simulink model "Zlinearyzowany"  (R2017a)
settings: Solver=FixedStepAuto  StartTime=0.0  StopTime=150  FixedStep=0.1  RelTol=1e-3  EnableMultiTasking=on
values from neighbouring files (symbols this model uses):
  A = pi*R1*R1    (= 10.9999393421)    [Lab2.m]    (also in ModelDataNonlinear.m)
  B = (pi*R2*R2)/(3*H2*H2)    (= 0.00337009933323)    [Lab2.m]    (also in Lab8.m = deltah20max / k; Lab9.m = 0.4; ModelDataNonlinear.m)
  C1 = 1.372    [Lab2.m]    (also in ModelDataNonlinear.m)
  C2 = 0.332756    [Lab2.m]    (also in ModelDataNonlinear.m)
  deltaw = deltaq1    [Lab2.m]    (also in Lab3.m = 0; Lab8.m = deltah20max / 3; ModelDataNonlinear.m = 0.1*w0)
  h10 = (q10/C1).^2    [Lab2.m]    (also in ModelDataNonlinear.m)
  h20 = h2max/2    (= 8)    [Lab2.m]    (also in ModelDataNonlinear.m)
  k = 5    [Lab1.m]    (also in Lab2.m = (2*sqrt(h20))/C2; ModelData.m = 17)
  kr = 1.84/2    (= 0.92)    [Lab1.m]    (also in Lab4.m = 0.95*T/(k*T0); Lab7.m = 0.0803; Lab9.m = 0.0679)
  q10 = C2*sqrt(h20)    [Lab2.m]    (also in ModelDataNonlinear.m)
  T1 = 3    [Lab1.m]    (also in Lab2.m = 2*pi*R1*R1*sqrt(h10)/C1; ModelData.m = 10.998)
  T2 = 4    [Lab1.m]    (also in Lab2.m = 2*A*sqrt(h10)/C1; ModelData.m = 10.998)
  T3 = 8    [Lab1.m]    (also in Lab3.m = 0.5*T1; Lab4.m = 0.5 * T1; ModelData.m = min(T1, T2) / 2)
  Td = 0.42*T0    [Lab4.m]
  Tf = 0.05 * Td    (= 0.19375)    [Lab4.m]
  Ti = 2.4*T0    [Lab4.m]    (also in Lab9.m = 17.823)
settings Model: Creator=Ganofir  LastModifiedBy=ishiguro
settings DataIOCC: SaveFormat=Array
settings OptimizationCC: LifeSpan=inf
settings DebuggingCC: ModelReferenceDataLoggingMessage=none  SFUnexpectedBacktrackingDiag=warning  SFNoUnconditionalDefaultTransitionDiag=warning  SFExecutionAtInitializationDiag=none
settings HardwareCC: ProdBitPerPointer=32  ProdBitPerSizeT=32  ProdBitPerPtrDiffT=32  ProdLargestAtomicFloat=None  ProdIntDivRoundTo=Undefined  ProdEndianess=Unspecified  ProdWordSize=32  ProdHWDeviceType=32-bit Generic
settings ModelReferenceCC: PropagateSignalLabelsOutOfModel=off
settings GRTTargetCC: TargetLangStandard=C89/C90 (ANSI)  GeneratePreprocessorConditionals=Disable all
settings ConfigComp: CovMetricSettings=dw  CovHtmlReporting=on  CovSaveCumulativeToWorkspaceVar=on  CovSaveSingleToWorkspaceVar=on  CovExternalEMLEnable=off

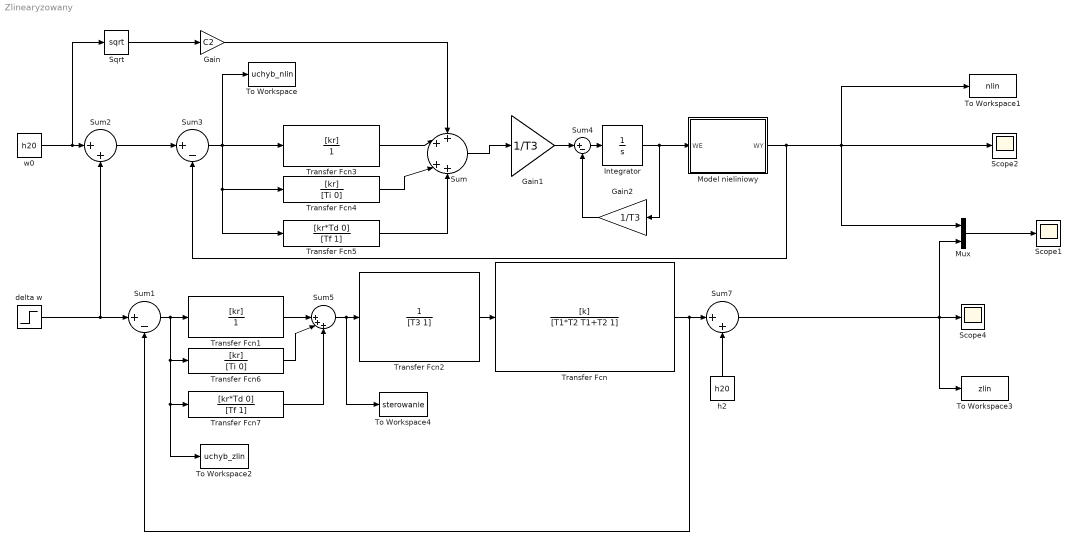
== system Zlinearyzowany ==
  Gain : Gain  Gain=C2
  Gain1 : Gain  Gain=1/T3
  Gain2 : Gain  Gain=1/T3
  Integrator : Integrator  InitialCondition=q10
  Model nieliniowy : Subsystem
  Mux : Mux  Inputs=2
  Scope1 : Scope
  Scope2 : Scope
  Scope4 : Scope
  Sqrt : Sqrt  SaturateOnIntegerOverflow=on
  Sum : Sum  Inputs=++|++
  Sum1 : Sum  Inputs=|+-
  Sum2 : Sum  Inputs=|++
  Sum3 : Sum  Inputs=|+-
  Sum4 : Sum  Inputs=|+-
  Sum5 : Sum  Inputs=||+++
  Sum7 : Sum  Inputs=|++
  To Workspace : ToWorkspace  VariableName=uchyb_nlin  SampleTime=-1
  To Workspace1 : ToWorkspace  VariableName=nlin  SampleTime=-1
  To Workspace2 : ToWorkspace  VariableName=uchyb_zlin  SampleTime=-1
  To Workspace3 : ToWorkspace  VariableName=zlin  SampleTime=-1
  To Workspace4 : ToWorkspace  VariableName=sterowanie  SampleTime=-1
  Transfer Fcn : TransferFcn  Numerator=[k]  Denominator=[T1*T2 T1+T2 1]
  Transfer Fcn1 : TransferFcn  Numerator=[kr]  Denominator=[1]
  Transfer Fcn2 : TransferFcn  Denominator=[T3 1]
  Transfer Fcn3 : TransferFcn  Numerator=[kr]  Denominator=[1]
  Transfer Fcn4 : TransferFcn  Numerator=[kr]  Denominator=[Ti 0]
  Transfer Fcn5 : TransferFcn  Numerator=[kr*Td 0]  Denominator=[Tf 1]
  Transfer Fcn6 : TransferFcn  Numerator=[kr]  Denominator=[Ti 0]
  Transfer Fcn7 : TransferFcn  Numerator=[kr*Td 0]  Denominator=[Tf 1]
  delta w : Step  Time=0  After=deltaw  SampleTime=0
  h2 : Constant  Value=h20
  w0 : Constant  Value=h20
  wires:
  delta w/1 -> Sum1/1, Sum2/2
  Sum7/1 -> Mux/2, To Workspace3/1, Scope4/1
  h2/1 -> Sum7/2
  Transfer Fcn/1 -> Sum1/2, Sum7/1
  Transfer Fcn2/1 -> Transfer Fcn/1
  Sum1/1 -> Transfer Fcn6/1, Transfer Fcn7/1, To Workspace2/1, Transfer Fcn1/1
  Mux/1 -> Scope1/1
  w0/1 -> Sqrt/1, Sum2/1
  Sum2/1 -> Sum3/1
  Sum3/1 -> Transfer Fcn4/1, Transfer Fcn5/1, To Workspace/1, Transfer Fcn3/1
  Integrator/1 -> Gain2/1, Model nieliniowy/1(WE)
  Model nieliniowy/1(WY) -> Sum3/2, To Workspace1/1, Scope2/1, Mux/1
  Sum/1 -> Gain1/1
  Transfer Fcn3/1 -> Sum/2
  Sqrt/1 -> Gain/1
  Gain/1 -> Sum/1
  Gain1/1 -> Sum4/1
  Sum4/1 -> Integrator/1
  Gain2/1 -> Sum4/2
  Transfer Fcn5/1 -> Sum/4
  Transfer Fcn4/1 -> Sum/3
  Transfer Fcn7/1 -> Sum5/3
  Transfer Fcn6/1 -> Sum5/2
  Transfer Fcn1/1 -> Sum5/1
  Sum5/1 -> To Workspace4/1, Transfer Fcn2/1

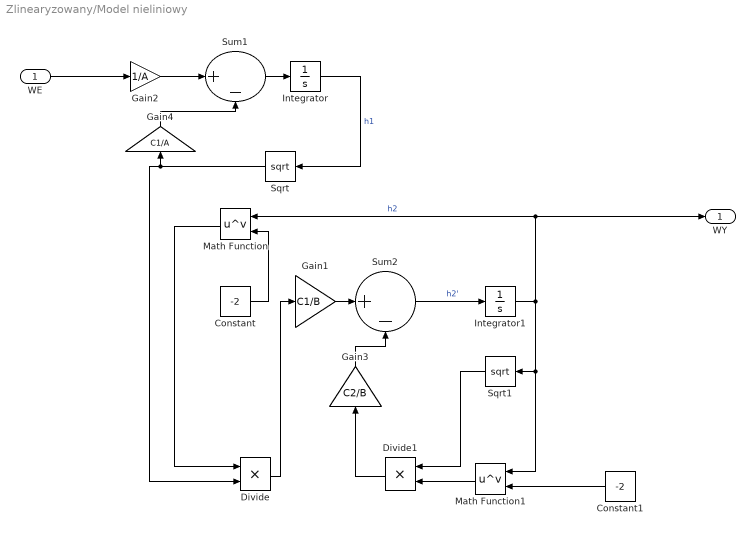
== system Zlinearyzowany/Model nieliniowy ==
  WE : Inport
  Constant : Constant  Value=-2
  Constant1 : Constant  Value=-2
  Divide : Product  Inputs=**
  Divide1 : Product  Inputs=**
  Gain1 : Gain  Gain=C1/B
  Gain2 : Gain  Gain=1/A
  Gain3 : Gain  Gain=C2/B
  Gain4 : Gain  Gain=C1/A
  Integrator : Integrator  InitialCondition=h10
  Integrator1 : Integrator  InitialCondition=h20
  Math Function : Math  Operator=pow  SaturateOnIntegerOverflow=on
  Math Function1 : Math  Operator=pow  SaturateOnIntegerOverflow=on
  Sqrt : Sqrt  SaturateOnIntegerOverflow=on
  Sqrt1 : Sqrt  SaturateOnIntegerOverflow=on
  Sum1 : Sum  Inputs=|+-
  Sum2 : Sum  Inputs=|+-
  WY : Outport
  wires:
  Sum1/1 -> Integrator/1
  Sqrt1/1 -> Divide1/1
  Gain4/1 -> Sum1/2
  Integrator1/1 -> Math Function/1, WY/1, Math Function1/1, Sqrt1/1  "h2"
  Sqrt/1 -> Divide/2, Gain4/1
  Gain3/1 -> Sum2/2
  Sum2/1 -> Integrator1/1  "h2'"
  Divide1/1 -> Gain3/1
  Integrator/1 -> Sqrt/1  "h1"
  Gain1/1 -> Sum2/1
  Divide/1 -> Gain1/1
  Gain2/1 -> Sum1/1
  WE/1 -> Gain2/1
  Constant/1 -> Math Function/2
  Math Function/1 -> Divide/1
  Math Function1/1 -> Divide1/2
  Constant1/1 -> Math Function1/2
